simulink model "bangbang"  (Simulink 6.0)
settings: Solver=ode23  SolverMode=SingleTasking  StartTime=0.0  StopTime=100  MaxStep=0.1  RelTol=1e-6  AbsTol=1e-6
settings Model: Creator=The MathWorks Inc.  LastModifiedBy=batserve  ExtModeAutoUpdateStatusClock=off
settings DataIOCC: ExternalInput=[]  InitialState=[]  LimitDataPoints=off  SaveOutput=off  SaveState=on  StateSaveName=x  TimeSaveName=t
settings DebuggingCC: CheckExecutionContextPreStartOutputMsg=on  CheckExecutionContextRuntimeOutputMsg=on  SolverPrmCheckMsg=none
settings HardwareCC: TargetUnknown=on

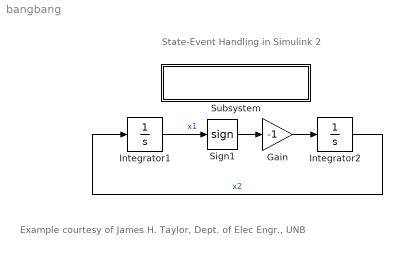
== system bangbang ==
  note: State-Event Handling in Simulink 2
  note: Example courtesy of James H. Taylor, Dept. of Elec Engr., UNB
  Gain : Gain  Gain=-1  SaturateOnIntegerOverflow=on
  Integrator1 : Integrator  InitialCondition=0.25
  Integrator2 : Integrator  InitialCondition=0.25
  Sign1 : Signum
  Subsystem : Subsystem  PropExecContextAcrossSSBoundary=on
      settings: DeleteFcn=if ishandle(get_param(gcbh,'UserData')),delete(get_param(gcbh,'UserData'));end  OpenFcn=if ~isempty(get_param(gcbh,'UserData')),if ishandle(get_param(gcbh,'UserData')),figure(get_param(gcbh,'UserData'));end;else,figure;end;[t,x]=sim(gcs);plot(x(:,1),x(:,2));shg;set_param(gcbh,'UserData',gcf)
      mask Display: fprintf('Double-Click\nto see a phase plane plot')
  wires:
  Integrator2/1 -> Integrator1/1  "x2"
  Integrator1/1 -> Sign1/1  "x1"
  Sign1/1 -> Gain/1
  Gain/1 -> Integrator2/1

== system bangbang/Subsystem ==
